simulink model "sparse_bayes_filter"  (R2021b)
settings: Solver=FixedStepAuto  StartTime=0.0  StopTime=100.0  FixedStep=0.01  RelTol=1e-3
libraries: wnnlib x26
settings Model: Creator=20214358  LastModifiedBy=20214358
settings HardwareCC: ProdLongLongMode=on  TargetBitPerPointer=64  TargetBitPerSizeT=64  TargetBitPerPtrDiffT=64  TargetLargestAtomicFloat=Float  TargetIntDivRoundTo=Zero  TargetEndianess=LittleEndian  TargetWordSize=64  TargetHWDeviceType=Intel->x86-64 (Windows64)

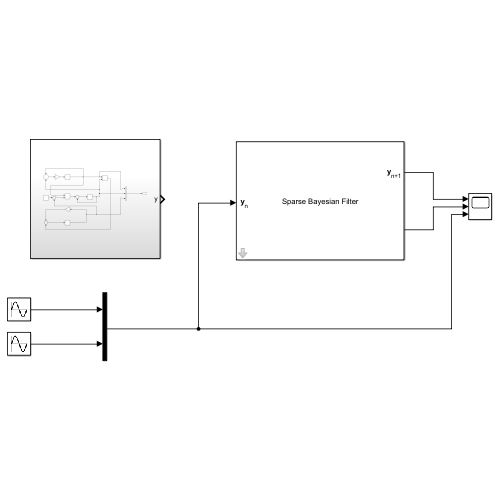
[thumbnail: Simulink's stored preview of the top-level diagram]
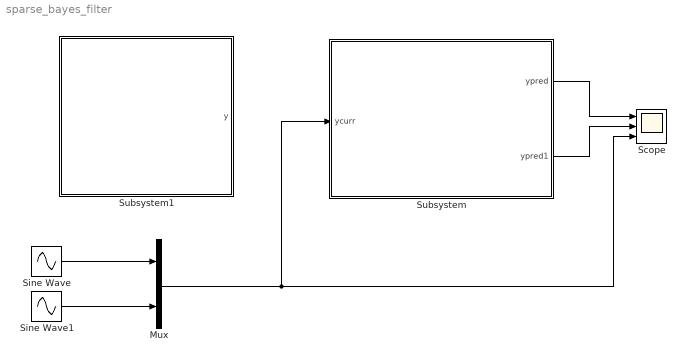
== system sparse_bayes_filter ==
  Mux : Mux  Inputs=2
  Scope : Scope  NumInputPorts=3
  Sine Wave : Sin  Amplitude=5  SampleTime=0
  Sine Wave1 : Sin  Amplitude=5  Phase=1  SampleTime=0
  Subsystem : Subsystem  mask{filter_match_tolerance=1, filter_number_of_random_flips=1, observation_dense_vector_length=2, observation_sparse_vector_length=2048, observation_memory_size=[511 512], observation_hamming_distance=[4 32], observation_vgram_array_length=16384, observation_number_of_samples=32, dynamics_memory_size=[511 512], dynamics_hamming_distance=[4 32], dynamics_vgram_array_length=4096, dynamics_number_of_samples=32, codec_number_of_sparse_vectors=16384, codec_learning_rate=0.0001, codec_min_bounds=[-10 -10], codec_max_bounds=[10 10], codec_sparse_vectors_file='C:\Users\20214358\MATLAB\Projects\wnnlib\wnndata\16k_sparse_vectors_seed_0.npz'}
      mask prompts: filter_match_tolerance "Match tolerance"; filter_number_of_random_flips "Number of random flips"; observation_dense_vector_length "Dense vector length"; observation_sparse_vector_length "Sparse vector length"; observation_memory_size "Memory size"; observation_hamming_distance "Hamming distance"; observation_vgram_array_length "VGRAM array length"; observation_number_of_samples "Number of samples"; dynamics_memory_size "Memory size"; dynamics_hamming_distance "Hamming distance"; dynamics_vgram_array_length "VGRAM array length"; dynamics_number_of_samples "Number of samples"; codec_number_of_sparse_vectors "Number of sparse vectors"; codec_learning_rate "Learning rate"; codec_min_bounds "Minimum bounds"; codec_max_bounds "Maximum bounds"; codec_sparse_vectors_file "Sparse vectors file"
      mask init:
      | codec_max_kdtree_depth = ceil(log2(codec_number_of_sparse_vectors));
      | codec_min_splitting_volume = prod(codec_max_bounds - codec_min_bounds)/codec_number_of_sparse_vectors;
      | codec_sparse_vectors_file = char(codec_sparse_vectors_file);
      mask DialogControl FilterParams Prompt: Filter
      mask DialogControl ObservationModelParams Prompt: Observation model
      mask DialogControl DynamicModelParams Prompt: Dynamic model
      mask DialogControl CodecParams Prompt: Codec
      mask Display:
      | disp('Sparse Bayesian Filter','interpreter','tex');
      | port_label('input', 1,'{\bf y}_{n}','interpreter','tex');
      | port_label('output', 1,'{\bf y}_{n+1}','interpreter','tex');
  Subsystem1 : Subsystem
  wires:
  Subsystem/1(ypred) -> Scope/1
  Mux/1 -> Subsystem/1(ycurr), Scope/3
  Sine Wave/1 -> Mux/1
  Sine Wave1/1 -> Mux/2
  Subsystem/2(ypred1) -> Scope/2

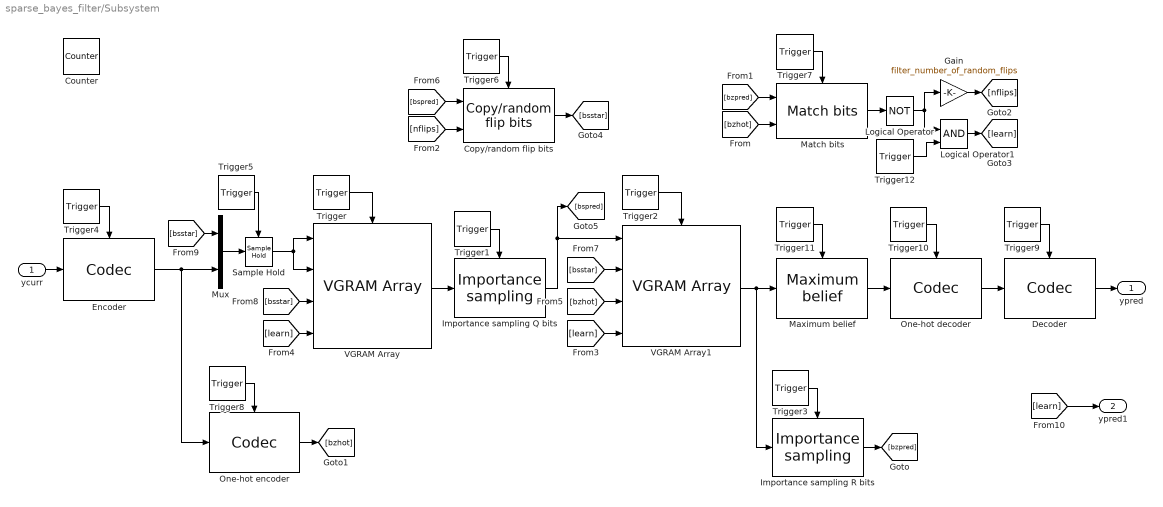
== system sparse_bayes_filter/Subsystem ==
  ycurr : Inport
  Copy/random flip bits : wnnlib/Utilities/Copy//random flip bits
      settings: SourceProductName=Weightless Neural Networks Toolbox
  Counter : wnnlib/Sources/Counter  number_of_steps=11  sample_time=-1
      settings: SourceProductName=Weightless Neural Networks Toolbox
  Decoder : wnnlib/Utilities/Codec  codec_id=0  dense_vector_length=observation_dense_vector_length  sparse_vector_length=observation_sparse_vector_length  max_depth=codec_max_kdtree_depth  learning_rate=codec_learning_rate  min_splitting_volume=codec_min_splitting_volume  min_bounds=codec_min_bounds  max_bounds=codec_max_bounds  sparse_vectors_file=codec_sparse_vectors_file  debug_flag=off  codec_type=Decoder  number_of_sparse_vectors=65536
      settings: SourceProductName=Weightless Neural Networks Toolbox
  Encoder : wnnlib/Utilities/Codec  codec_id=0  dense_vector_length=observation_dense_vector_length  sparse_vector_length=observation_sparse_vector_length  max_depth=codec_max_kdtree_depth  learning_rate=codec_learning_rate  min_splitting_volume=codec_min_splitting_volume  min_bounds=codec_min_bounds  max_bounds=codec_max_bounds  sparse_vectors_file=codec_sparse_vectors_file  debug_flag=on  codec_type=Encoder  number_of_sparse_vectors=65536
      settings: SourceProductName=Weightless Neural Networks Toolbox
  Gain : Gain  Gain=filter_number_of_random_flips  OutDataTypeStr=uint8
  Importance sampling Q bits : wnnlib/Utilities/Importance sampling  nSamples=dynamics_number_of_samples
      settings: SourceProductName=Weightless Neural Networks Toolbox
  Importance sampling R bits : wnnlib/Utilities/Importance sampling  nSamples=observation_number_of_samples
      settings: SourceProductName=Weightless Neural Networks Toolbox
  Logical Operator : Logic  Operator=NOT  IconShape=distinctive  AllPortsSameDT=off  OutDataTypeStr=boolean
  Logical Operator1 : Logic  IconShape=distinctive  AllPortsSameDT=off  OutDataTypeStr=boolean
  Match bits : wnnlib/Utilities/Match bits  nMatchTolerance=filter_match_tolerance
      settings: SourceProductName=Weightless Neural Networks Toolbox
  Maximum belief : wnnlib/Utilities/Maximum belief  SystemSampleTime=-1  VariantActivationTime=update diagram  Latency=0  AutoFrameSizeCalculation=off
      settings: SourceProductName=Weightless Neural Networks Toolbox
  Mux : Mux  Inputs=2
  One-hot decoder : wnnlib/Utilities/Codec  codec_id=0  dense_vector_length=observation_dense_vector_length  sparse_vector_length=observation_sparse_vector_length  max_depth=codec_max_kdtree_depth  learning_rate=codec_learning_rate  min_splitting_volume=codec_min_splitting_volume  min_bounds=codec_min_bounds  max_bounds=codec_max_bounds  sparse_vectors_file=codec_sparse_vectors_file  debug_flag=off  codec_type=OneHotDecoder  number_of_sparse_vectors=codec_number_of_sparse_vectors
      settings: SourceProductName=Weightless Neural Networks Toolbox
  One-hot encoder : wnnlib/Utilities/Codec  codec_id=0  dense_vector_length=observation_dense_vector_length  sparse_vector_length=observation_sparse_vector_length  max_depth=codec_max_kdtree_depth  learning_rate=codec_learning_rate  min_splitting_volume=codec_min_splitting_volume  min_bounds=codec_min_bounds  max_bounds=codec_max_bounds  sparse_vectors_file=codec_sparse_vectors_file  debug_flag=off  codec_type=OneHotEncoder  number_of_sparse_vectors=codec_number_of_sparse_vectors
      settings: SourceProductName=Weightless Neural Networks Toolbox
  Sample Hold : wnnlib/Utilities/Sample Hold  sample_time=-1
      settings: SourceProductName=Weightless Neural Networks Toolbox
  Trigger : wnnlib/Sources/Trigger  selected_steps=[2 8]
      settings: SourceProductName=Weightless Neural Networks Toolbox
  Trigger1 : wnnlib/Sources/Trigger  selected_steps=[3 9]
      settings: SourceProductName=Weightless Neural Networks Toolbox
  Trigger10 : wnnlib/Sources/Trigger  selected_steps=[6 10]
      settings: SourceProductName=Weightless Neural Networks Toolbox
  Trigger11 : wnnlib/Sources/Trigger  selected_steps=[5 9]
      settings: SourceProductName=Weightless Neural Networks Toolbox
  Trigger12 : wnnlib/Sources/Trigger  selected_steps=7
      settings: SourceProductName=Weightless Neural Networks Toolbox
  Trigger2 : wnnlib/Sources/Trigger  selected_steps=[2 8]
      settings: SourceProductName=Weightless Neural Networks Toolbox
  Trigger3 : wnnlib/Sources/Trigger  selected_steps=5
      settings: SourceProductName=Weightless Neural Networks Toolbox
  Trigger4 : wnnlib/Sources/Trigger  selected_steps=0
      settings: SourceProductName=Weightless Neural Networks Toolbox
  Trigger5 : wnnlib/Sources/Trigger  selected_steps=11
      settings: SourceProductName=Weightless Neural Networks Toolbox
  Trigger6 : wnnlib/Sources/Trigger  selected_steps=[7 10]
      settings: SourceProductName=Weightless Neural Networks Toolbox
  Trigger7 : wnnlib/Sources/Trigger  selected_steps=6
      settings: SourceProductName=Weightless Neural Networks Toolbox
  Trigger8 : wnnlib/Sources/Trigger  selected_steps=1
      settings: SourceProductName=Weightless Neural Networks Toolbox
  Trigger9 : wnnlib/Sources/Trigger  selected_steps=[7 11]
      settings: SourceProductName=Weightless Neural Networks Toolbox
  VGRAM Array : wnnlib/Models/VGRAM Array  array_id=0  min_mem_size=dynamics_memory_size(1)  max_mem_size=dynamics_memory_size(2)  min_dist=dynamics_hamming_distance(1)  max_dist=dynamics_hamming_distance(2)  pattern_length=dynamics_vgram_array_length+observation_sparse_vector_length  output_dims=[dynamics_vgram_array_length 1]  debug_flag=off
      settings: SourceProductName=Weightless Neural Networks Toolbox
  VGRAM Array1 : wnnlib/Models/VGRAM Array  array_id=1  min_mem_size=observation_memory_size(1)  max_mem_size=observation_memory_size(2)  min_dist=observation_hamming_distance(1)  max_dist=observation_hamming_distance(2)  pattern_length=dynamics_vgram_array_length  output_dims=[observation_vgram_array_length 1]  debug_flag=on
      settings: SourceProductName=Weightless Neural Networks Toolbox
  ypred : Outport
  ypred1 : Outport  Port=2
  wires:
  Trigger1/1 -> Importance sampling Q bits/Trigger
  ycurr/1 -> Encoder/1
  Trigger2/1 -> VGRAM Array1/Trigger
  VGRAM Array/1 -> Importance sampling Q bits/1
  Importance sampling Q bits/1 -> [bspred], VGRAM Array1/1
  Trigger4/1 -> Encoder/Trigger
  Trigger7/1 -> Match bits/Trigger
  Trigger6/1 -> Copy/random flip bits/Trigger
  Match bits/1 -> Logical Operator/1
  Trigger/1 -> VGRAM Array/Trigger
  [bzhot] -> Match bits/2
  Trigger5/1 -> Sample Hold/Trigger
  Trigger3/1 -> Importance sampling R bits/Trigger
  [bzpred] -> Match bits/1
  Logical Operator/1 -> Logical Operator1/1, Gain/1
  [nflips] -> Copy/random flip bits/2
  Gain/1 -> [nflips]
  Importance sampling R bits/1 -> [bzpred]
  [bsstar] -> VGRAM Array/3
  Trigger8/1 -> One-hot encoder/Trigger
  One-hot encoder/1 -> [bzhot]
  [bzhot] -> VGRAM Array1/3
  [bspred] -> Copy/random flip bits/1
  Copy/random flip bits/1 -> [bsstar]
  [bsstar] -> VGRAM Array1/2
  Decoder/1 -> ypred/1
  Trigger9/1 -> Decoder/Trigger
  Mux/1 -> Sample Hold/1
  [bsstar] -> Mux/1
  One-hot decoder/1 -> Decoder/1
  Trigger10/1 -> One-hot decoder/Trigger
  Trigger11/1 -> Maximum belief/Trigger
  Trigger12/1 -> Logical Operator1/2
  Encoder/1 -> Mux/2, One-hot encoder/1
  Sample Hold/1 -> VGRAM Array/2, VGRAM Array/1
  Logical Operator1/1 -> [learn]
  [learn] -> VGRAM Array1/4
  VGRAM Array1/1 -> Maximum belief/1, Importance sampling R bits/1
  [learn] -> VGRAM Array/4
  Maximum belief/1 -> One-hot decoder/1
  [learn] -> ypred1/1

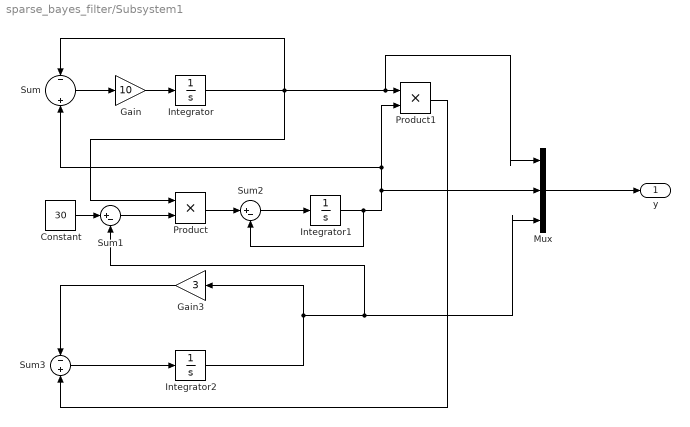
== system sparse_bayes_filter/Subsystem1 ==
  Constant : Constant  Value=30
  Gain : Gain  Gain=10
  Gain3 : Gain  Gain=3
  Integrator : Integrator  InitialCondition=5
  Integrator1 : Integrator  InitialCondition=5
  Integrator2 : Integrator  InitialCondition=5
  Mux : Mux  Inputs=3
  Product : Product
  Product1 : Product
  Sum : Sum  Inputs=-|||+
  Sum1 : Sum  Inputs=|+-
  Sum2 : Sum  Inputs=|+-
  Sum3 : Sum  Inputs=-+
  y : Outport
  wires:
  Constant/1 -> Sum1/1
  Integrator2/1 -> Gain3/1, Mux/3, Sum1/2
  Product/1 -> Sum2/1
  Integrator1/1 -> Sum2/2, Mux/2, Product1/2, Sum/2
  Gain3/1 -> Sum3/1
  Sum3/1 -> Integrator2/1
  Sum2/1 -> Integrator1/1
  Sum1/1 -> Product/2
  Gain/1 -> Integrator/1
  Sum/1 -> Gain/1
  Product1/1 -> Sum3/2
  Integrator/1 -> Mux/1, Product1/1, Product/1, Sum/1
  Mux/1 -> y/1
